simulink subsystem "DCDC_plant_model"  (R2021a)
settings: Solver=VariableStepAuto  StartTime=0.0  StopTime=10.0  RelTol=1e-3
undefined symbols (not defined in the file): CarrierResolution, CarrierTime, DeadTime, Init_time, sensCutoff_Freq, SimulationTimeStep
libraries: fl_lib x14, nesl_utility x9, simulink x1
settings Model: Creator=tshintai  LastModifiedBy=tshintai
settings SolverCC: AlgebraicLoopSolver=TrustRegion
settings DebuggingCC: SFMachineParentedDataDiag=warning

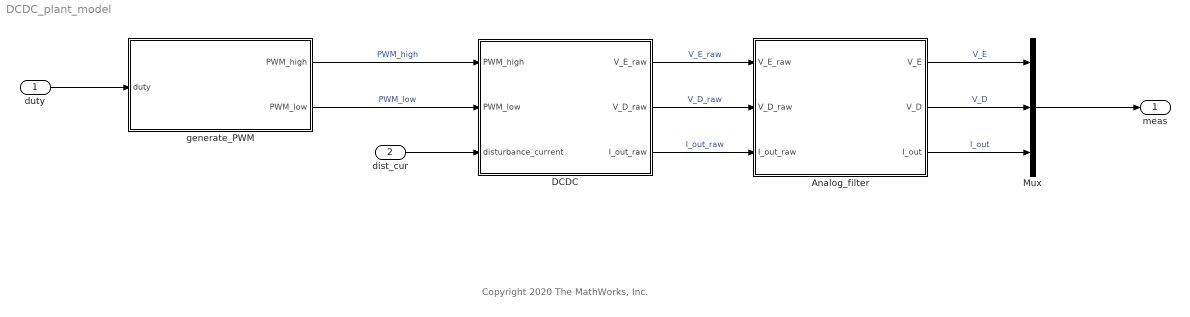
== system DCDC_plant_model ==
  note: Copyright 2020 The MathWorks, Inc.
  duty : Inport
  dist_cur : Inport  Port=2
  Analog_filter : Subsystem
  DCDC : Subsystem
  Mux : Mux  Inputs=3
  generate_PWM : Subsystem
  meas : Outport  VectorParamsAs1DForOutWhenUnconnected=off
  wires:
  duty/1 -> generate_PWM/1(duty)
  generate_PWM/1(PWM_high) -> DCDC/1(PWM_high)  "PWM_high"
  generate_PWM/2(PWM_low) -> DCDC/2(PWM_low)  "PWM_low"
  DCDC/1(V_E_raw) -> Analog_filter/1(V_E_raw)  "V_E_raw"
  DCDC/2(V_D_raw) -> Analog_filter/2(V_D_raw)  "V_D_raw"
  DCDC/3(I_out_raw) -> Analog_filter/3(I_out_raw)  "I_out_raw"
  Mux/1 -> meas/1
  Analog_filter/2(V_D) -> Mux/2  "V_D"
  Analog_filter/1(V_E) -> Mux/1  "V_E"
  Analog_filter/3(I_out) -> Mux/3  "I_out"
  dist_cur/1 -> DCDC/3(disturbance_current)

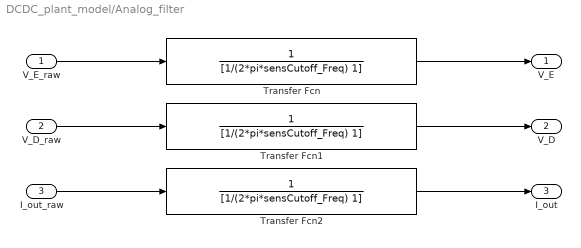
== system DCDC_plant_model/Analog_filter ==
  V_E_raw : Inport
  V_D_raw : Inport  Port=2
  I_out_raw : Inport  Port=3
  Transfer Fcn : TransferFcn  Denominator=[1/(2*pi*sensCutoff_Freq) 1]
  Transfer Fcn1 : TransferFcn  Denominator=[1/(2*pi*sensCutoff_Freq) 1]
  Transfer Fcn2 : TransferFcn  Denominator=[1/(2*pi*sensCutoff_Freq) 1]
  V_E : Outport
  V_D : Outport  Port=2
  I_out : Outport  Port=3
  wires:
  Transfer Fcn2/1 -> I_out/1
  Transfer Fcn1/1 -> V_D/1
  I_out_raw/1 -> Transfer Fcn2/1
  V_E_raw/1 -> Transfer Fcn/1
  Transfer Fcn/1 -> V_E/1
  V_D_raw/1 -> Transfer Fcn1/1

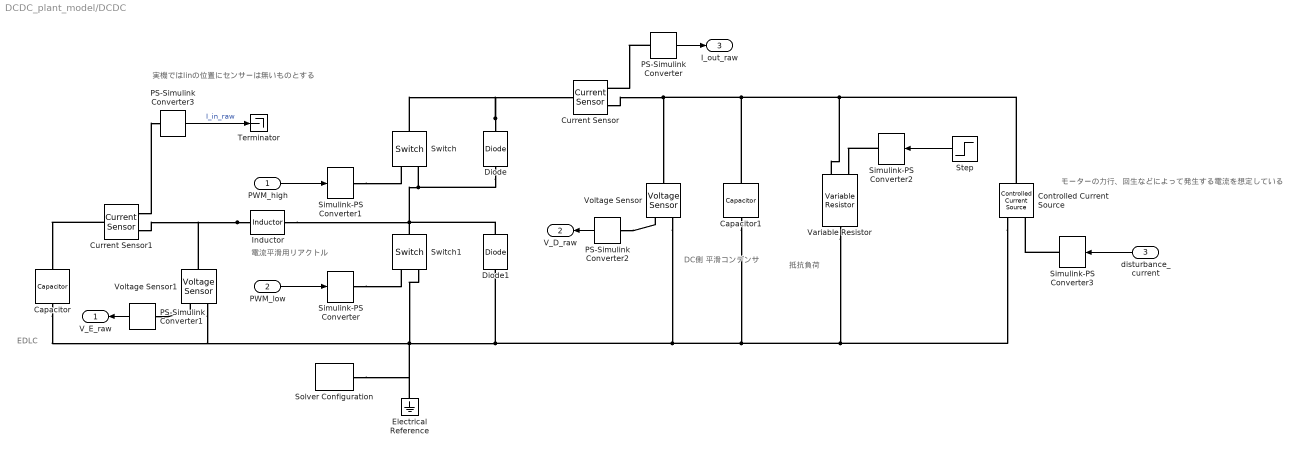
== system DCDC_plant_model/DCDC ==
  note: 実機ではIinの位置にセンサーは無いものとする
  note: EDLC
  note: 抵抗負荷
  note: DC側
      | 平滑コンデンサ
  note: 電流平滑用リアクトル
  note: モーターの力行、回生などによって発生する電流を想定している
  PWM_high : Inport
  PWM_low : Inport  Port=2
  disturbance_current : Inport  Port=3
  Capacitor : fl_lib/Electrical/Electrical Elements/Capacitor  c=EDLC_Capacitance F  r=EDLC_internal_R Ohm  g=0 1/Ohm  i_specify=off  i_priority=High  i=0 A  i_nominal_specify=off  i_nominal_unit=A  i_nominal_value=1  v_specify=off  v_priority=None  v=0 V  v_nominal_specify=off  v_nominal_unit=V  v_nominal_value=1  vc_specify=on  vc_priority=High  vc=EDLC_InitialVoltage V  vc_nominal_specify=off  vc_nominal_unit=V  vc_nominal_value=1
  Capacitor1 : fl_lib/Electrical/Electrical Elements/Capacitor  c=DC_Capacitance F  r=0.51 Ohm  g=0 1/Ohm  i_specify=off  i_priority=High  i=0 A  i_nominal_specify=off  i_nominal_unit=A  i_nominal_value=1  v_specify=off  v_priority=None  v=0 V  v_nominal_specify=off  v_nominal_unit=V  v_nominal_value=1  vc_specify=on  vc_priority=High  vc=DC_InitialVoltage V  vc_nominal_specify=off  vc_nominal_unit=V  vc_nominal_value=1
  Controlled Current Source : fl_lib/Electrical/Electrical Sources/Controlled Current Source
  Current Sensor : fl_lib/Electrical/Electrical Sensors/Current Sensor
  Current Sensor1 : fl_lib/Electrical/Electrical Sensors/Current Sensor
  Diode : fl_lib/Electrical/Electrical Elements/Diode  Vf=0.6 V  Ron=0.3 Ohm  Goff=1e-8 1/Ohm  i_specify=off  i_priority=High  i=0 A  i_nominal_specify=off  i_nominal_unit=A  i_nominal_value=1  v_specify=off  v_priority=High  v=0 V  v_nominal_specify=off  v_nominal_unit=V  v_nominal_value=1
  Diode1 : fl_lib/Electrical/Electrical Elements/Diode  Vf=0.6 V  Ron=0.3 Ohm  Goff=1e-8 1/Ohm  i_specify=off  i_priority=High  i=0 A  i_nominal_specify=off  i_nominal_unit=A  i_nominal_value=1  v_specify=off  v_priority=High  v=0 V  v_nominal_specify=off  v_nominal_unit=V  v_nominal_value=1
  Electrical Reference : fl_lib/Electrical/Electrical Elements/Electrical Reference
  Inductor : fl_lib/Electrical/Electrical Elements/Inductor  l=Reactance H  r=0.05 Ohm  g=1e-9 1/Ohm  i_specify=on  i_priority=Low  i=0 A  i_nominal_specify=off  i_nominal_unit=A  i_nominal_value=1  v_specify=on  v_priority=Low  v=0 V  v_nominal_specify=off  v_nominal_unit=V  v_nominal_value=1  i_L_specify=off  i_L_priority=High  i_L=0 A  i_L_nominal_specify=off  i_L_nominal_unit=A  i_L_nominal_value=1
  PS-Simulink Converter{,1..3} (4 alike) : nesl_utility/PS-Simulink Converter  PhysicalDomain=network_engine_domain  SubClassName=ps_output  LeftPortType=input  RightPortType=output  PseudoPeriodic=off  Frequencies=[]  Unit=1  AffineConversion=off
      settings: SourceProductBaseCode=PW,SS
  Simulink-PS Converter{,1..3} (4 alike) : nesl_utility/Simulink-PS Converter  PhysicalDomain=network_engine_domain  SubClassName=ps_input  LeftPortType=input  RightPortType=output  PseudoPeriodic=off  Frequencies=[]  NoiseDistribution=none  NoiseParameters=[]  Unit=1  AffineConversion=off  FilteringAndDerivatives=zero  SimscapeFilterOrder=1  InputFilterTimeConstant=0.001  UdotUserProvided=1
      settings: SourceProductBaseCode=PW,SS
  Solver Configuration : nesl_utility/Solver Configuration  PhysicalDomain=network_engine_domain  SubClassName=solver  LeftPortType=input  RightPortType=generic  Tones=[]  Harmonics=[]  SimulateNoise=off  Profile=off  UseLocalSampling=off  EnableSwitchedLinearOptims=on  FrequencyDomain=off  UseCCode=off  RelTol=0.001  AbsTol=1e-06  MinStep=1e-09  ToWorkspace=off  RevertToSquareIcSolve=off  NumHomotopyIterations=100  PhasorMode=off  PhasorModeNumHarmonics=1  DoDC=off  ResidualTolerance=1e-09  UseLocalSolver=on  LocalSolverChoice=NE_BACKWARD_EULER_ADVANCER  LocalSolverSampleTime=SimulationTimeStep  DoFixedCost=on  MaxNonlinIter=3  MaxModeIter=2  ComputeImpulses=off  ImpulseIterations=2  LinearAlgebra=Sparse  EquationFormulation=NE_TIME_EF  DelaysMemoryBudget=1024  AutomaticFiltering=off  FilteringTimeConstant=0.001  PartitionStorageMethod=AS_NEEDED  PartitionMemoryBudget=1024  PartitionMethod=FAST
      settings: SourceProductBaseCode=PW,SS
  Step : Step  Time=0.1  Before=160 / 0.001  After=160 / 0.001  SampleTime=SimulationTimeStep
  Switch : fl_lib/Electrical/Electrical Elements/Switch  R_closed=0.01 Ohm  G_open=1e-8 1/Ohm  Threshold=0.5  i_specify=off  i_priority=High  i=0 A  i_nominal_specify=off  i_nominal_unit=A  i_nominal_value=1  v_specify=off  v_priority=High  v=0 V  v_nominal_specify=off  v_nominal_unit=V  v_nominal_value=1
  Switch1 : fl_lib/Electrical/Electrical Elements/Switch  R_closed=0.01 Ohm  G_open=1e-8 1/Ohm  Threshold=0.5  i_specify=off  i_priority=High  i=0 A  i_nominal_specify=off  i_nominal_unit=A  i_nominal_value=1  v_specify=off  v_priority=High  v=0 V  v_nominal_specify=off  v_nominal_unit=V  v_nominal_value=1
  Terminator : Terminator
  Variable Resistor : fl_lib/Electrical/Electrical Elements/Variable Resistor  Rmin=0 Ohm  i_specify=off  i_priority=High  i=0 A  i_nominal_specify=off  i_nominal_unit=A  i_nominal_value=1  v_specify=off  v_priority=High  v=0 V  v_nominal_specify=off  v_nominal_unit=V  v_nominal_value=1
  Voltage Sensor : fl_lib/Electrical/Electrical Sensors/Voltage Sensor
  Voltage Sensor1 : fl_lib/Electrical/Electrical Sensors/Voltage Sensor
  V_E_raw : Outport  VectorParamsAs1DForOutWhenUnconnected=off
  V_D_raw : Outport  Port=2  VectorParamsAs1DForOutWhenUnconnected=off
  I_out_raw : Outport  Port=3  VectorParamsAs1DForOutWhenUnconnected=off
  wires:
  disturbance_current/1 -> Simulink-PS Converter3/1
  Step/1 -> Simulink-PS Converter2/1
  PS-Simulink Converter3/1 -> Terminator/1  "I_in_raw"
  PS-Simulink Converter/1 -> I_out_raw/1
  PWM_high/1 -> Simulink-PS Converter1/1
  PS-Simulink Converter1/1 -> V_E_raw/1
  PWM_low/1 -> Simulink-PS Converter/1
  PS-Simulink Converter2/1 -> V_D_raw/1
  connections:
  Simulink-PS Converter3/RConn1 -- Controlled Current Source/RConn1
  Inductor/LConn1 -- Current Sensor1/RConn2 -- Voltage Sensor1/LConn1
  PS-Simulink Converter/LConn1 -- Current Sensor/RConn1
  Current Sensor1/LConn1 -- Capacitor/LConn1
  PS-Simulink Converter1/LConn1 -- Voltage Sensor1/RConn1
  Simulink-PS Converter/RConn1 -- Switch1/RConn1
  Current Sensor1/RConn1 -- PS-Simulink Converter3/LConn1
  Simulink-PS Converter2/RConn1 -- Variable Resistor/LConn1
  Diode1/RConn1 -- Inductor/RConn1 -- Switch1/LConn1 -- Diode/LConn1 -- Switch/RConn2
  PS-Simulink Converter2/LConn1 -- Voltage Sensor/RConn1
  Diode/RConn1 -- Current Sensor/LConn1 -- Switch/LConn1
  Simulink-PS Converter1/RConn1 -- Switch/RConn1
  Controlled Current Source/RConn2 -- Variable Resistor/RConn1 -- Capacitor1/RConn1 -- Voltage Sensor/RConn2 -- Solver Configuration/RConn1 -- Electrical Reference/LConn1 -- Capacitor/RConn1 -- Voltage Sensor1/RConn2 -- Switch1/RConn2 -- Diode1/LConn1
  Controlled Current Source/LConn1 -- Variable Resistor/LConn2 -- Capacitor1/LConn1 -- Voltage Sensor/LConn1 -- Current Sensor/RConn2

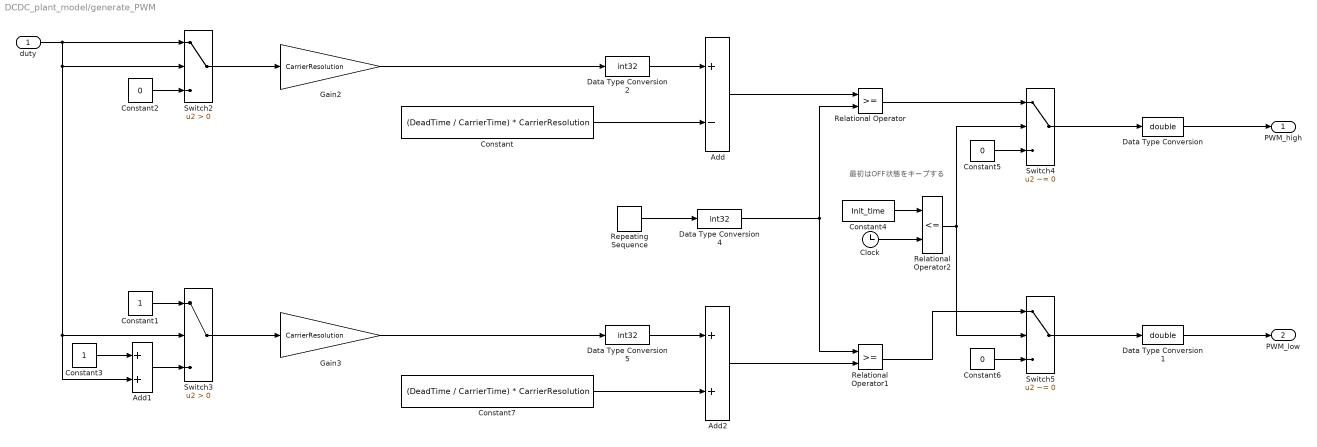
== system DCDC_plant_model/generate_PWM ==
  note: 最初はOFF状態をキープする
  duty : Inport
  Add : Sum  Inputs=+-
  Add1 : Sum
  Add2 : Sum
  Clock : Clock
  Constant : Constant  Value=(DeadTime / CarrierTime) * CarrierResolution  OutDataTypeStr=int32
  Constant1 : Constant
  Constant2 : Constant  Value=0
  Constant3 : Constant
  Constant4 : Constant  Value=Init_time
  Constant5 : Constant  Value=0  OutDataTypeStr=boolean
  Constant6 : Constant  Value=0  OutDataTypeStr=boolean
  Constant7 : Constant  Value=(DeadTime / CarrierTime) * CarrierResolution  OutDataTypeStr=int32
  Data Type Conversion : DataTypeConversion  OutDataTypeStr=double
  Data Type Conversion1 : DataTypeConversion  OutDataTypeStr=double
  Data Type Conversion2 : DataTypeConversion  OutDataTypeStr=int32  RndMeth=Nearest
      settings: AttributesFormatString=丸め方向 = %<RndMeth>
  Data Type Conversion4 : DataTypeConversion  OutDataTypeStr=int32  RndMeth=Nearest
      settings: AttributesFormatString=丸め方向 = %<RndMeth>
  Data Type Conversion5 : DataTypeConversion  OutDataTypeStr=int32  RndMeth=Nearest
      settings: AttributesFormatString=丸め方向 = %<RndMeth>
  Gain2 : Gain  Gain=CarrierResolution
  Gain3 : Gain  Gain=CarrierResolution
  Relational Operator : RelationalOperator  OutDataTypeStr=boolean  RndMeth=Nearest
  Relational Operator1 : RelationalOperator  OutDataTypeStr=boolean  RndMeth=Nearest
  Relational Operator2 : RelationalOperator  Operator=<=  OutDataTypeStr=boolean  RndMeth=Nearest
  Repeating Sequence : simulink/Sources/Repeating Sequence  rep_seq_t=[0, CarrierTime / 2, CarrierTime]  rep_seq_y=[0, CarrierResolution, 0]
  Switch2 : Switch  Criteria=u2 > Threshold
  Switch3 : Switch  Criteria=u2 > Threshold
  Switch4 : Switch  Criteria=u2 ~= 0
  Switch5 : Switch  Criteria=u2 ~= 0
  PWM_high : Outport
  PWM_low : Outport  Port=2
  wires:
  Add1/1 -> Switch3/3
  Constant/1 -> Add/2
  Data Type Conversion4/1 -> Relational Operator1/1, Relational Operator/2
  Data Type Conversion2/1 -> Add/1
  Constant2/1 -> Switch2/3
  Constant4/1 -> Relational Operator2/1
  Relational Operator1/1 -> Switch5/1
  Constant7/1 -> Add2/2
  Data Type Conversion1/1 -> PWM_low/1
  Gain2/1 -> Data Type Conversion2/1
  Relational Operator/1 -> Switch4/1
  Add2/1 -> Relational Operator1/2
  Data Type Conversion/1 -> PWM_high/1
  Constant5/1 -> Switch4/3
  duty/1 -> Add1/2, Switch3/2, Switch2/2, Switch2/1
  Gain3/1 -> Data Type Conversion5/1
  Switch5/1 -> Data Type Conversion1/1
  Data Type Conversion5/1 -> Add2/1
  Clock/1 -> Relational Operator2/2
  Switch2/1 -> Gain2/1
  Add/1 -> Relational Operator/1
  Constant1/1 -> Switch3/1
  Repeating Sequence/1 -> Data Type Conversion4/1
  Switch3/1 -> Gain3/1
  Constant3/1 -> Add1/1
  Switch4/1 -> Data Type Conversion/1
  Constant6/1 -> Switch5/3
  Relational Operator2/1 -> Switch4/2, Switch5/2
